simulink model "robotics"  (R2019b)
settings: Solver=VariableStepAuto  StartTime=0.0  StopTime=5  RelTol=1e-3
settings Model: Creator=ADMIN  LastModifiedBy=ADMIN

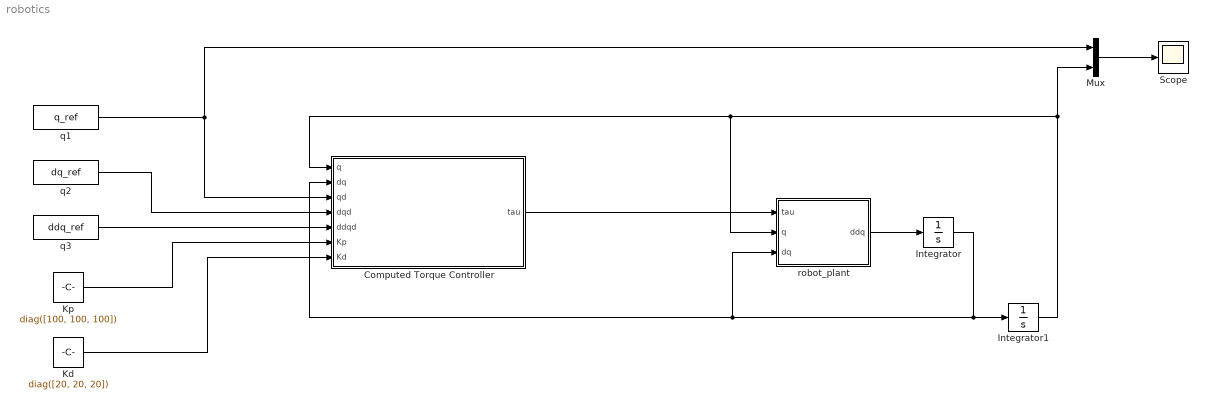
== system robotics ==
  Computed Torque Controller : MATLAB Function  TreatAsAtomicUnit=on
  Integrator : Integrator  InitialCondition=[0; 0; 0]
  Integrator1 : Integrator  InitialCondition=[0; 0.17; 0]
  Kd : Constant  Value=diag([20, 20, 20])
  Kp : Constant  Value=diag([100, 100, 100])
  Mux : Mux  Inputs=2
  Scope : Scope
  q1 : FromWorkspace  VariableName=q_ref  SampleTime=0
  q2 : FromWorkspace  VariableName=dq_ref  SampleTime=0
  q3 : FromWorkspace  VariableName=ddq_ref  SampleTime=0
  robot_plant : MATLAB Function  TreatAsAtomicUnit=on
  wires:
  robot_plant/1(ddq) -> Integrator/1
  Integrator/1 -> Computed Torque Controller/2(dq), robot_plant/3(dq), Integrator1/1
  Integrator1/1 -> Mux/2, robot_plant/2(q), Computed Torque Controller/1(q)
  Computed Torque Controller/1(tau) -> robot_plant/1(tau)
  Kp/1 -> Computed Torque Controller/6(Kp)
  Kd/1 -> Computed Torque Controller/7(Kd)
  q1/1 -> Mux/1, Computed Torque Controller/3(qd)
  q2/1 -> Computed Torque Controller/4(dqd)
  q3/1 -> Computed Torque Controller/5(ddqd)
  Mux/1 -> Scope/1

== matlab function robotics/Computed Torque Controller ==
  data: q input; tau output; dq input; qd input; dqd input; ddqd input; Kp input; Kd input
function tau = controller( q, dq, qd, dqd, ddqd, Kp, Kd)
       % Luật điều khiển ngẫu lực tính toán
       M = calc_M(q);
       C = calc_C(q, dq);
       G = calc_G(q);
       
       tau = M * (ddqd + Kd*(dqd - dq) + Kp*(qd - q)) + C*dq + G;
   end

== matlab function robotics/robot_plant ==
  data: tau input; ddq output; q input; dq input
function ddq = robot_plant(tau, q, dq)
    % Tính toán gia tốc khớp từ momen đầu vào
    M = calc_M(q);
    C = calc_C(q, dq);
    G = calc_G(q);

    ddq = M \ (tau - C*dq - G);
end
